simulink model "task2"  (R2022b)
settings: Solver=FixedStepAuto  StartTime=0.0  StopTime=7  RelTol=1e-8
undefined symbols (not defined in the file): a0, A1, a1, a2, A3, b0, B1, b1, b2, B3, C1, C3
settings Model: Creator=anton  LastModifiedBy=anton
settings DataIOCC: ExternalInput=data  LoadExternalInput=on

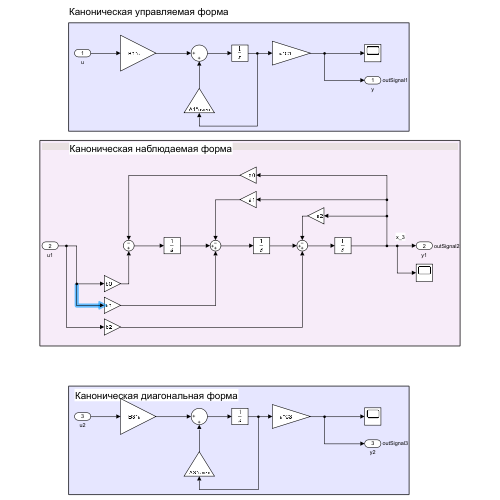
[thumbnail: Simulink's stored preview of the top-level diagram]
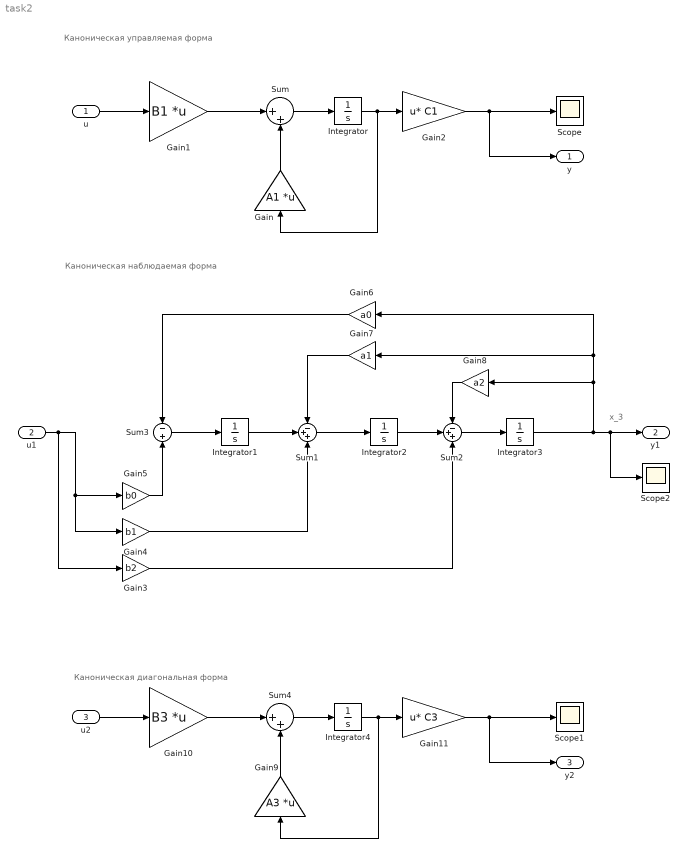
== system task2 ==
  note: x_3
  note: Каноническая управляемая форма
  note: Каноническая наблюдаемая форма
  note: Каноническая диагональная форма
  u : Inport  PortDimensions=1
  u1 : Inport  Port=2  PortDimensions=1
  u2 : Inport  Port=3  PortDimensions=1
  Gain : Gain  Gain=A1  Multiplication=Matrix(K*u) (u vector)
  Gain1 : Gain  Gain=B1  Multiplication=Matrix(K*u)
  Gain10 : Gain  Gain=B3  Multiplication=Matrix(K*u)
  Gain11 : Gain  Gain=C3  Multiplication=Matrix(u*K)
  Gain2 : Gain  Gain=C1  Multiplication=Matrix(u*K)
  Gain3 : Gain  Gain=b2
  Gain4 : Gain  Gain=b1
  Gain5 : Gain  Gain=b0
  Gain6 : Gain  Gain=a0
  Gain7 : Gain  Gain=a1
  Gain8 : Gain  Gain=a2
  Gain9 : Gain  Gain=A3  Multiplication=Matrix(K*u) (u vector)
  Integrator{,1..4} (5 alike) : Integrator
  Scope : Scope
  Scope1 : Scope
  Scope2 : Scope
  Sum : Sum  Inputs=|++
  Sum1 : Sum  Inputs=-++
  Sum2 : Sum  Inputs=-++
  Sum3 : Sum  Inputs=-+
  Sum4 : Sum  Inputs=|++
  y : Outport  SignalName=outSignal1
  y1 : Outport  Port=2  SignalName=outSignal2
  y2 : Outport  Port=3  SignalName=outSignal3
  wires:
  u/1 -> Gain1/1
  Gain1/1 -> Sum/1
  Sum/1 -> Integrator/1
  Gain/1 -> Sum/2
  Integrator/1 -> Gain/1, Gain2/1
  Gain2/1 -> y/1, Scope/1
  u1/1 -> Gain3/1, Gain4/1, Gain5/1
  Integrator3/1 -> Scope2/1, y1/1, Gain7/1, Gain6/1, Gain8/1
  Gain5/1 -> Sum3/2
  Gain6/1 -> Sum3/1
  Sum3/1 -> Integrator1/1
  Sum1/1 -> Integrator2/1
  Integrator1/1 -> Sum1/2
  Gain7/1 -> Sum1/1
  Integrator2/1 -> Sum2/2
  Sum2/1 -> Integrator3/1
  Gain4/1 -> Sum1/3
  Gain3/1 -> Sum2/3
  Gain8/1 -> Sum2/1
  Sum4/1 -> Integrator4/1
  u2/1 -> Gain10/1
  Gain10/1 -> Sum4/1
  Integrator4/1 -> Gain9/1, Gain11/1
  Gain11/1 -> y2/1, Scope1/1
  Gain9/1 -> Sum4/2
